simulink model "pdmDeterioratingSystemEstimation"  (R2022a)
settings: Solver=FixedStepDiscrete  StartTime=0.0  StopTime=200  RelTol=1e-3  EnableMultiTasking=on
PreLoadFcn:
  | Ts = 1/256;
  | ynoi = 0.2;
  | num0 = [1     -0.10075     -0.26052     -0.24022];
  | den0 = [1      -4.5049       8.2675      -7.7122       3.6508         -0.7];
  | numF = [1.2642     -0.12736     -0.32935     -0.30369];
  | denF = [1      -4.5674        8.511      -8.0697       3.8856     -0.75805];
  | PFnum = [0.00034    0.0017652   -0.0013829];
  | PFden = [1       -1.896      0.91629];
StartFcn:
  | clear idARMAXSpectrumPlot
values from neighbouring files (symbols this model uses):
  initial_model = translatecov(@(x)idpoly(x),model)    [Fault_Detect_DataBasedModels.m]
undefined symbols (not defined in the file or in its folder): getcov
libraries: slident x1
CloseFcn:
  | close(gcf)
settings Model: Creator=The MathWorks, Inc.  LastModifiedBy=The MathWorks, Inc.
settings SolverCC: AlgebraicLoopSolver=TrustRegion  MinimalZcImpactIntegration=on
settings DataIOCC: LimitDataPoints=on  ReturnWorkspaceOutputs=off
settings OptimizationCC: LifeSpan=inf
settings DebuggingCC: UnconnectedInputMsg=warning  UnconnectedOutputMsg=warning  UnconnectedLineMsg=warning  AllowSymbolicDim=off  SFUnexpectedBacktrackingDiag=warning  SFNoUnconditionalDefaultTransitionDiag=warning  SFExecutionAtInitializationDiag=none  SFMachineParentedDataDiag=warning  ArithmeticOperatorsInVariantConditions=warning
settings HardwareCC: ProdBitPerPointer=32  ProdBitPerSizeT=32  ProdBitPerPtrDiffT=32  ProdLargestAtomicFloat=None  ProdIntDivRoundTo=Undefined  ProdEndianess=Unspecified  ProdWordSize=32  ProdHWDeviceType=32-bit Generic
settings ModelReferenceCC: PropagateSignalLabelsOutOfModel=off
settings SFSimCC: SimUseLocalCustomCode=off  CustomCodeUndefinedFunction=UseInterfaceOnly
settings RTWCC: RTWUseLocalCustomCode=off  DLArmComputeVersion=19.05
settings CodeAppCC: StateflowObjectComments=on
settings GRTTargetCC: TargetLangStandard=C89/C90 (ANSI)
settings ConfigComp: CovMetricSettings=dw  CovSaveCumulativeToWorkspaceVar=on  CovSaveSingleToWorkspaceVar=on  CovExternalEMLEnable=off

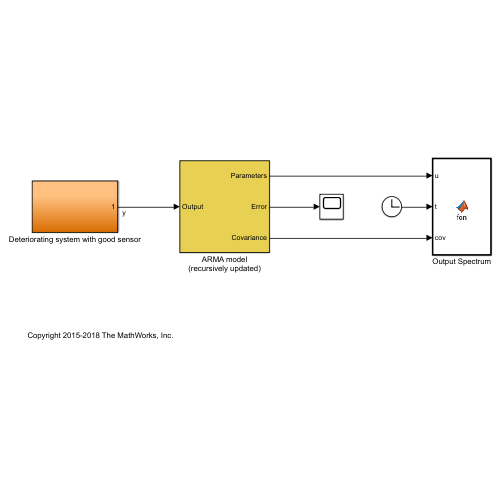
[thumbnail: Simulink's stored preview of the top-level diagram]
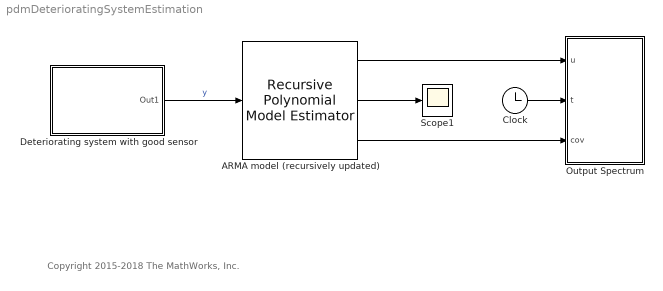
== system pdmDeterioratingSystemEstimation ==
  note: Copyright 2015-2018 The MathWorks, Inc.
  ARMA model (recursively updated) : slident/Estimators/Recursive Polynomial Model Estimator  ModelStructure=ARMA  InitialEstimateSource=Internal  A0=initial_model.a  B0=1  C0=initial_model.c  D0=1  F0=1  nk=1  P0=getcov(initial_model )  InitialInputs=0  InitialOutputs=0  History=Infinite  WindowLength=200  EstimationMethod=Forgetting Factor  AdaptationParameter=0.9997  HasTimeVaryingAdaptationParameter=off  NormalizationBias=eps  OutputError=on  OutputP=on  AddEnablePort=off  InputProcessing=Sample-based  Ts=Ts
      settings: SourceProductBaseCode=ID
  Clock : Clock
  Deteriorating system with good sensor : Subsystem  VariantControl=DeterioratingSystem
  Output Spectrum : MATLAB Function
  Scope1 : Scope
  wires:
  Deteriorating system with good sensor/1(Out1) -> ARMA model (recursively updated)/1  "y"
  ARMA model (recursively updated)/1 -> Output Spectrum/1(u)
  ARMA model (recursively updated)/3 -> Output Spectrum/3(cov)
  Clock/1 -> Output Spectrum/2(t)
  ARMA model (recursively updated)/2 -> Scope1/1

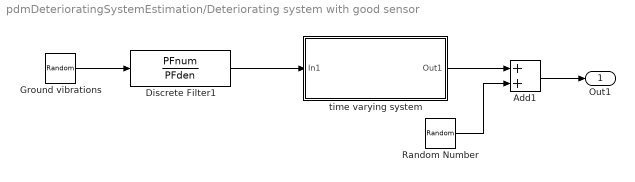
== system pdmDeterioratingSystemEstimation/Deteriorating system with good sensor ==
  Add1 : Sum
  Discrete Filter1 : DiscreteFilter  Numerator=PFnum  Denominator=PFden
  Ground vibrations : RandomNumber  Variance=0.62074  SampleTime=Ts
  Random Number : RandomNumber  Variance=ynoi  SampleTime=Ts
  time varying system : Subsystem
  Out1 : Outport  VectorParamsAs1DForOutWhenUnconnected=off
  wires:
  Random Number/1 -> Add1/2
  Add1/1 -> Out1/1
  Ground vibrations/1 -> Discrete Filter1/1
  time varying system/1(Out1) -> Add1/1
  Discrete Filter1/1 -> time varying system/1(In1)

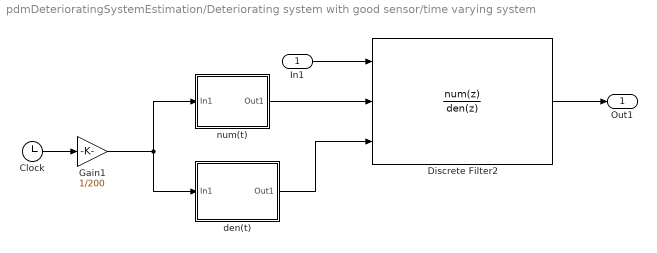
== system pdmDeterioratingSystemEstimation/Deteriorating system with good sensor/time varying system ==
  In1 : Inport
  Clock : Clock
  Discrete Filter2 : DiscreteFilter  NumeratorSource=Input port  Numerator=PFnum  DenominatorSource=Input port  Denominator=PFden  a0EqualsOne=on
      settings: InputPortMap=u0,p1,p3
  Gain1 : Gain  Gain=1/200
  den(t) : Subsystem
  num(t) : Subsystem
  Out1 : Outport  VectorParamsAs1DForOutWhenUnconnected=off
  wires:
  Clock/1 -> Gain1/1
  Gain1/1 -> den(t)/1(In1), num(t)/1(In1)
  In1/1 -> Discrete Filter2/1
  Discrete Filter2/1 -> Out1/1
  num(t)/1(Out1) -> Discrete Filter2/2
  den(t)/1(Out1) -> Discrete Filter2/3

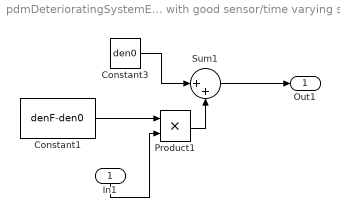
== system pdmDeterioratingSystemEstimation/Deteriorating system with good sensor/time varying system/den(t) ==
  In1 : Inport  SampleTime=Ts
  Constant1 : Constant  Value=denF-den0  SampleTime=Ts
  Constant3 : Constant  Value=den0  SampleTime=Ts
  Product1 : Product
  Sum1 : Sum  Inputs=|++
  Out1 : Outport  VectorParamsAs1DForOutWhenUnconnected=off
  wires:
  In1/1 -> Product1/2
  Sum1/1 -> Out1/1
  Constant3/1 -> Sum1/1
  Product1/1 -> Sum1/2
  Constant1/1 -> Product1/1

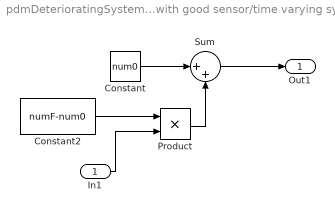
== system pdmDeterioratingSystemEstimation/Deteriorating system with good sensor/time varying system/num(t) ==
  In1 : Inport  SampleTime=Ts
  Constant : Constant  Value=num0  SampleTime=Ts
  Constant2 : Constant  Value=numF-num0  SampleTime=Ts
  Product : Product
  Sum : Sum  Inputs=|++
  Out1 : Outport  VectorParamsAs1DForOutWhenUnconnected=off
  wires:
  In1/1 -> Product/2
  Constant/1 -> Sum/1
  Sum/1 -> Out1/1
  Constant2/1 -> Product/1
  Product/1 -> Sum/2

== matlab function pdmDeterioratingSystemEstimation/Output Spectrum ==
  data: u input; t input; cov input
function fcn(u,t,cov)
% Code for the Output Spectrum block.

coder.extrinsic('pdmARMASpectrumPlot')
l = 8;
a = u(1:l);
c = u(l+1:end-1);

pdmARMASpectrumPlot(a, c, t, cov)
